simulink model "TestFlightSim1D_g"  (R2020b)
settings: Solver=VariableStepAuto  StartTime=0.0  StopTime=80  RelTol=1e-10
settings Model: Creator=jonathan  LastModifiedBy=jonathan

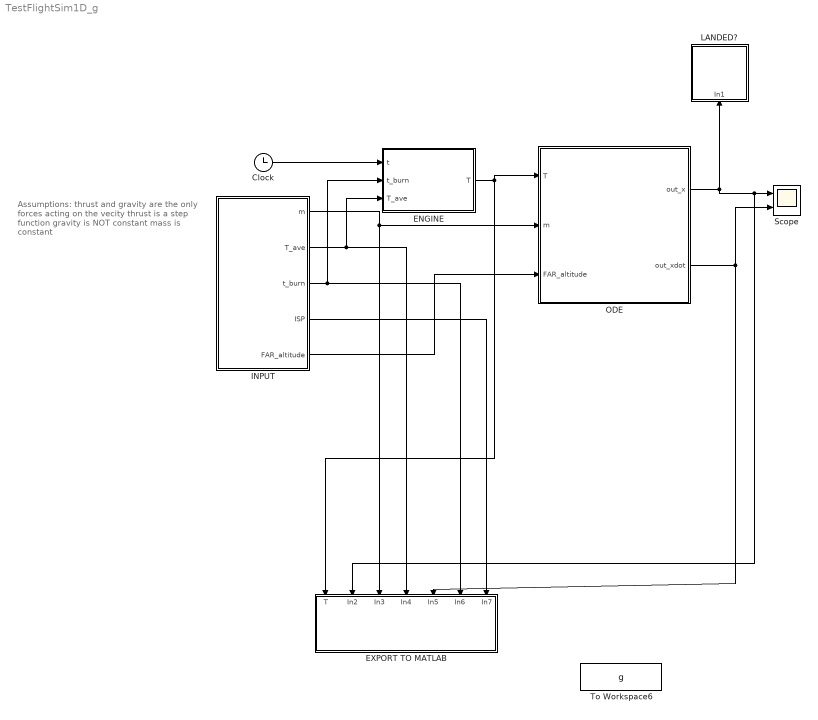
== system TestFlightSim1D_g ==
  note: Assumptions:
      | thrust and gravity are the only forces acting on the vecity
      | thrust is a step function
      | gravity is NOT constant
      | mass is constant
  Clock : Clock
  ENGINE : MATLAB Function  TreatAsAtomicUnit=on
  EXPORT TO MATLAB : Subsystem
  INPUT : MATLAB Function  TreatAsAtomicUnit=on
  LANDED? : Subsystem
  ODE : Subsystem
  Scope : Scope  NumInputPorts=2
  To Workspace6 : ToWorkspace  VariableName=g  SaveFormat=Timeseries  SampleTime=-1
  wires:
  Clock/1 -> ENGINE/1(t)
  INPUT/2(T_ave) -> EXPORT TO MATLAB/4(In4), ENGINE/3(T_ave)
  INPUT/3(t_burn) -> EXPORT TO MATLAB/6(In6), ENGINE/2(t_burn)
  INPUT/1(m) -> EXPORT TO MATLAB/3(In3), ODE/2(m)
  ODE/2(out_xdot) -> Scope/2, EXPORT TO MATLAB/5(In5)
  ODE/1(out_x) -> LANDED?/1(In1), Scope/1, EXPORT TO MATLAB/2(In2)
  ENGINE/1(T) -> EXPORT TO MATLAB/1(T), ODE/1(T)
  ? -> To Workspace6/1
  INPUT/4(ISP) -> EXPORT TO MATLAB/7(In7)
  INPUT/5(FAR_altitude) -> ODE/3(FAR_altitude)

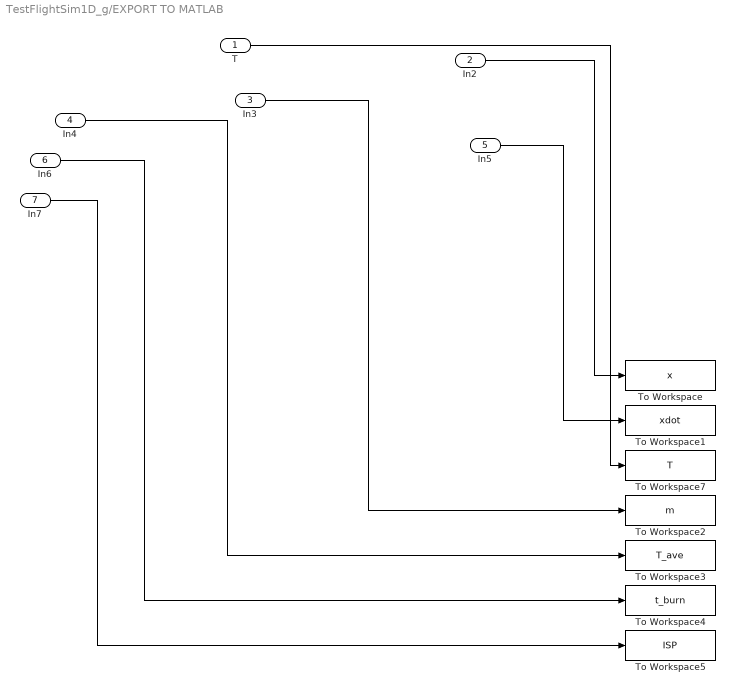
== system TestFlightSim1D_g/EXPORT TO MATLAB ==
  T : Inport
  In2 : Inport  Port=2
  In3 : Inport  Port=3
  In4 : Inport  Port=4
  In5 : Inport  Port=5
  In6 : Inport  Port=6
  In7 : Inport  Port=7
  To Workspace : ToWorkspace  VariableName=x  SaveFormat=Timeseries  SampleTime=-1
  To Workspace1 : ToWorkspace  VariableName=xdot  SaveFormat=Timeseries  SampleTime=-1
  To Workspace2 : ToWorkspace  VariableName=m  SaveFormat=Timeseries  SampleTime=-1
  To Workspace3 : ToWorkspace  VariableName=T_ave  SaveFormat=Timeseries  SampleTime=-1
  To Workspace4 : ToWorkspace  VariableName=t_burn  SaveFormat=Timeseries  SampleTime=-1
  To Workspace5 : ToWorkspace  VariableName=ISP  SaveFormat=Timeseries  SampleTime=-1
  To Workspace7 : ToWorkspace  VariableName=T  SaveFormat=Timeseries  SampleTime=-1
  wires:
  In6/1 -> To Workspace4/1
  In5/1 -> To Workspace1/1
  In7/1 -> To Workspace5/1
  In4/1 -> To Workspace3/1
  T/1 -> To Workspace7/1
  In2/1 -> To Workspace/1
  In3/1 -> To Workspace2/1

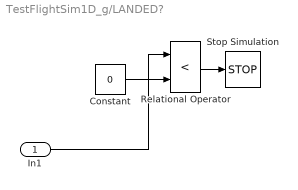
== system TestFlightSim1D_g/LANDED? ==
  In1 : Inport
  Constant : Constant  Value=0
  Relational Operator : RelationalOperator  Operator=<  OutDataTypeStr=boolean  RndMeth=Simplest
  Stop Simulation : Stop
  wires:
  In1/1 -> Relational Operator/1
  Constant/1 -> Relational Operator/2
  Relational Operator/1 -> Stop Simulation/1

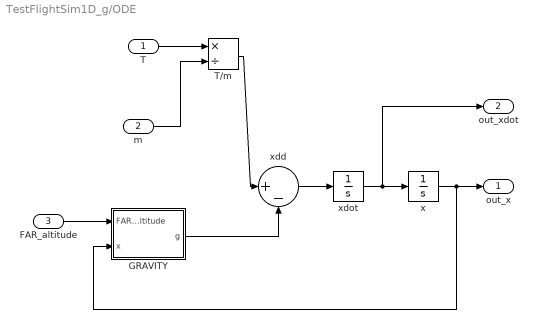
== system TestFlightSim1D_g/ODE ==
  T : Inport
  m : Inport  Port=2
  FAR_altitude : Inport  Port=3
  GRAVITY : MATLAB Function  TreatAsAtomicUnit=on
  T/m : Product  Inputs=*/
  x : Integrator
  xdd : Sum  Inputs=|+-
  xdot : Integrator
  out_x : Outport
  out_xdot : Outport  Port=2
  wires:
  m/1 -> T/m/2
  T/1 -> T/m/1
  x/1 -> GRAVITY/2(x), out_x/1
  xdot/1 -> out_xdot/1, x/1
  T/m/1 -> xdd/1
  xdd/1 -> xdot/1
  FAR_altitude/1 -> GRAVITY/1(FAR_altitude)
  GRAVITY/1(g) -> xdd/2

== matlab function TestFlightSim1D_g/ENGINE ==
  data: t input; t_burn input; T output; T_ave input
function T = fcn(t,t_burn,T_ave)
if t < t_burn
    T = T_ave;
else
    T = 0;
end
end

== matlab function TestFlightSim1D_g/INPUT ==
  data: m output; T_ave output; t_burn output; ISP output; FAR_altitude output
function [m,T_ave,t_burn,ISP,FAR_altitude] = fcn
% m - vehicle mass (assumed constant)
% m_fuel - fuel mass
% T_ave - average thrust
% ISP - specific impulse of engine
% FAR_altitude - altitude at FAR

m = 90; % [kg]
m_fuel = 16; % [kg]
T_ave = 3900; % [N]
ISP = 230; % [kg]
FAR_altitude = 1068.0192; % [m] altitude of Ransburg, CA

% calculate burntime
t_burn = ISP*9.8*m_fuel/T_ave;

end

== matlab function TestFlightSim1D_g/ODE/GRAVITY ==
  data: FAR_altitude input; g output; x input
function g = fcn(FAR_altitude,x)

RE = 6378e3; % [m] earth sea level radius
Mu_E = 3.986e14; % [m3/s2] gravitational parameter of earth

r = RE + FAR_altitude + x;

g = Mu_E*r^(-2);

end
